simulink model "redundancy"  (R2020b)
settings: Solver=ode15s  StartTime=0.0  StopTime=T  MaxStep=0.01  RelTol=1e-3
values from neighbouring files (symbols this model uses):
  a1A = L1    (= 0.35)    [forward_kinematics_computation.m]
  a1B = L1    (= 0.35)    [forward_kinematics_computation.m]
  a2A = L2    (= 0.305)    [forward_kinematics_computation.m]
  a2B = L2    (= 0.305)    [forward_kinematics_computation.m]
  a3A = L3    (= 0.2662)    [forward_kinematics_computation.m]
  a3B = L3    (= 0.2662)    [forward_kinematics_computation.m]
  D = 1.047    [forward_kinematics_computation.m]
  dq0 = [0 0 0 0 0 0]'    [sim_redundancy.m]
  friction = [fv1p fv2p fv1A fv2A fv3A fv1B fv2B fv3B]    [sim_redundancy.m]
  g = [0 -g0 0]'    [sim_redundancy.m]
  Gd = diag([1000 1000 1000 1000 1000])    [sim_redundancy.m]
  Gd_nullspace = 10*eye(6)    [sim_redundancy.m]
  Gp = diag([3000 3000 3000 3000 1000])    [sim_redundancy.m]
  Gp_nullspace = 10*eye(6)    [sim_redundancy.m]
  info = struct('n_joints', n_joints,                'n_links', n_links,                'n_ee', n_ee,                'current_frame_index',    [1  2 3 4 5 6 7  8 9 10],                'previous_frame_index',   [0  1 2 3 4 2 6  7 5  8],                'next_frame_index',       [2 36 4 5 9 7 8 10 0  0],                'next_frame_type',        [0  1 0 0 0 0 0  0 0  0],                'previous_joint_index',  ...(+449 chars)    [sim_redundancy.m]
  Kd = 20*eye(6)    [sim_redundancy.m]
  Kp = 10*eye(6)    [sim_redundancy.m]
  L = 3.16 + 0.126    (= 3.286)    [forward_kinematics_computation.m]
  l1A = a1A/2    (= 0.175)    [forward_kinematics_computation.m]
  l1B = a1B/2    (= 0.175)    [forward_kinematics_computation.m]
  l2A = a2A/2    (= 0.1525)    [forward_kinematics_computation.m]
  l2B = a2B/2    (= 0.1525)    [forward_kinematics_computation.m]
  l3A = a3A/2    (= 0.1331)    [forward_kinematics_computation.m]
  l3B = a3B/2    (= 0.1331)    [forward_kinematics_computation.m]
  offA = -0.19    [forward_kinematics_computation.m]
  offB = 0.19    [forward_kinematics_computation.m]
  prova = 2    [sim_redundancy.m]
  q0 = [th1A_0 th2A_0 th3A_0 th1B_0 th2B_0 th3B_0]'    [sim_redundancy.m]
  qr = [0 -pi/3 pi/4 0 pi/4 pi/8]    [sim_redundancy.m]
  qr_ddot = zeros(1,6)    [sim_redundancy.m]
  qr_dot = zeros(1,6)    [sim_redundancy.m]
  th1A_0 = -pi/6    (= -0.523598775598)    [sim_redundancy.m]
  th1B_0 = pi/6    (= 0.523598775598)    [sim_redundancy.m]
  th2A_0 = pi/6    (= 0.523598775598)    [sim_redundancy.m]
  th2B_0 = -pi/6    (= -0.523598775598)    [sim_redundancy.m]
  th3A_0 = pi/6    (= 0.523598775598)    [sim_redundancy.m]
  th3B_0 = -pi/6    (= -0.523598775598)    [sim_redundancy.m]
  tipo_controllo = 1    [sim_redundancy.m]
  tipo_minimizzazione = 4    [sim_redundancy.m]
  x_ref = [-0.25 -0.8 0.19 -0.9 0]    [sim_redundancy.m]
  xddot_ref = [0 0 0 0 0]    [sim_redundancy.m]
  xdot_ref = [0 0 0 0 0]    [sim_redundancy.m]
undefined symbols (not defined in the file or in its folder): fv0, fv1A, fv1B, fv2A, fv2B, fv3A, fv3B, g0, Il1Azz, Il1Bzz, Il2Azz, Il2Bzz, Il3Azz, Il3Bzz, m_cables, m_crane, m_platform, ml1A, ml1B, ml2A, ml2B, ml3A, ml3B, X, Y, Z
libraries: sm_lib x137, nesl_utility x31
(part 1 of 5)
settings Model: Creator=giank  LastModifiedBy=giank
settings ExplorerConfigSet: InternalSimMechanicsExplorerSettings="<ExplorerConfiguration><canonicalview>default</canonicalview><AnimationSetting><BasePlaybackSpeed>1.0</BasePlaybackSpeed><PlaybackSpeedFactor>4.0</PlaybackSpeedFactor></AnimationSetting><TilePanel><TileInfo><Tiles Columns=\"1\" Count=\"1\" Rows=\"1\"><Column Weight=\"1\"/><Row Weight=\"1\"/><Tile Height=\"1\" Width=\"1\" X=\"0\" Y=\"0\"/></Tiles></TileInfo><SceneInfo><SceneViewer><BGColor><R>0.60000002384185791</R><G>0.60000002384185791</G><B>0.60000002384185791</B></BGColor><Camera><DoPerspective>off</DoPerspective><Position><X>8.32344120016426103e-09</X><Y>-2.30749996473441854</Y><Z>2.62102653220962445</Z></Position><Center><X>8.32344120016426103e-09</X><Y>-2.30749996473441854</Y><Z>6.6162316514351005e-08</Z></Center><Up><X>0</X><Y>1</Y><Z>-0</Z></Up><ViewLimDist>1</ViewLimDist><YLim>2.35612490177154532</YLim><XLim>3.05834251955443737</XLim></Camera></SceneViewer></SceneInfo></TilePanel><MechEditorPanel><Cameras/><GfxPanelCameraMap/><VideoCreator><PlaybackSpeedRatio>1.0</PlaybackSpeedRatio><FrameRate>30</FrameRate><VideoFormat>Motion JPEG AVI</VideoFormat><FrameSize>auto</FrameSize></VideoCreator></MechEditorPanel></ExplorerConfiguration>"

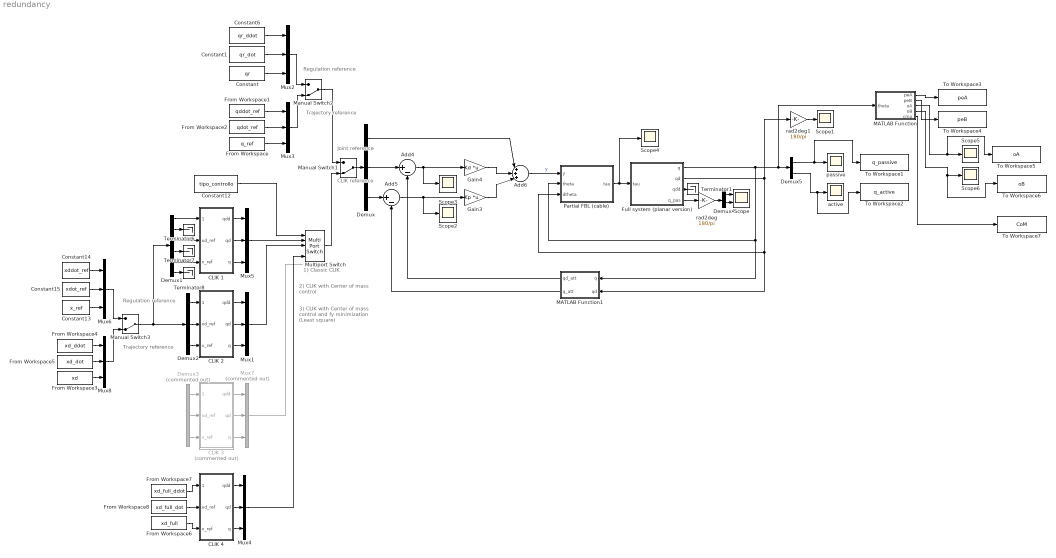
== system redundancy ==
  note: Regulation
      | reference
  note: CLIK
      | reference
  note: Trajectory
      | reference
  note: 3) CLIK with
      | Center of mass
      | control and
      | fy minimization
      | (Least square)
  note: 1) Classic
      | CLIK
  note: Trajectory
      | reference
  note: 2) CLIK with
      | Center of mass
      | control
  note: Joint
      | reference
  note: Regulation
      | reference
  Add4 : Sum  Inputs=|+-
  Add5 : Sum  Inputs=|+-
  Add6 : Sum  Inputs=|+++|
  CLIK 1 : Subsystem
  CLIK 2 : Subsystem
  CLIK 3 : Subsystem  Commented=on
  CLIK 4 : Subsystem
  Constant : Constant  Value=qr
  Constant1 : Constant  Value=qr_dot
  Constant12 : Constant  Value=tipo_controllo
  Constant13 : Constant  Value=x_ref
  Constant14 : Constant  Value=xddot_ref
  Constant15 : Constant  Value=xdot_ref
  Constant6 : Constant  Value=qr_ddot
  Demux : Demux  Outputs=3
  Demux1 : Demux  Outputs=[4 1 4 1 4 1]
  Demux2 : Demux  Outputs=[5 5 5]
  Demux3 : Demux  Commented=on  Outputs=[5 5 5]
  Demux4 : Demux  Outputs=2
  Demux5 : Demux  Outputs=[2 6]
  From Workspace : FromWorkspace  VariableName=q_ref
  From Workspace1 : FromWorkspace  VariableName=qddot_ref
  From Workspace2 : FromWorkspace  VariableName=qdot_ref
  From Workspace3 : FromWorkspace  VariableName=xd
  From Workspace4 : FromWorkspace  VariableName=xd_ddot
  From Workspace5 : FromWorkspace  VariableName=xd_dot
  From Workspace6 : FromWorkspace  VariableName=xd_full
  From Workspace7 : FromWorkspace  VariableName=xd_full_ddot
  From Workspace8 : FromWorkspace  VariableName=xd_full_dot
  Full system (planar version) : Subsystem
  Gain3 : Gain  Gain=Kp  Multiplication=Matrix(K*u)
  Gain4 : Gain  Gain=Kd  Multiplication=Matrix(K*u)
  MATLAB Function : MATLAB Function  TreatAsAtomicUnit=on
  MATLAB Function1 : MATLAB Function  TreatAsAtomicUnit=on
  Manual Switch1 : ManualSwitch  CurrentSetting=0
  Manual Switch2 : ManualSwitch  CurrentSetting=0
  Manual Switch3 : ManualSwitch  CurrentSetting=0
  Multiport Switch : MultiPortSwitch  DataPortOrder=Specify indices  DataPortIndices={1,2,3,4}
  Mux{1..6,8} (7 alike) : Mux  Inputs=3
  Mux7 : Mux  Commented=on  Inputs=3
  Partial FBL (cable) : MATLAB Function  TreatAsAtomicUnit=on
  Scope : Scope  NumInputPorts=2
  Scope{1..6} (6 alike) : Scope
  Terminator{1,6..8} (4 alike) : Terminator
  To Workspace1 : ToWorkspace  VariableName=q_passive  SaveFormat=Timeseries  SampleTime=-1
  To Workspace2 : ToWorkspace  VariableName=q_active  SaveFormat=Timeseries  SampleTime=-1
  To Workspace3 : ToWorkspace  VariableName=peA  SaveFormat=Timeseries  SampleTime=-1
  To Workspace4 : ToWorkspace  VariableName=peB  SaveFormat=Timeseries  SampleTime=-1
  To Workspace5 : ToWorkspace  VariableName=oA  SaveFormat=Timeseries  SampleTime=-1
  To Workspace6 : ToWorkspace  VariableName=oB  SaveFormat=Timeseries  SampleTime=-1
  To Workspace7 : ToWorkspace  VariableName=CoM  SaveFormat=Timeseries  SampleTime=-1
  active : Scope
  passive : Scope
  rad2deg : Gain  Gain=180/pi
  rad2deg1 : Gain  Gain=180/pi
  wires:
  Gain3/1 -> Add6/3
  Add6/1 -> Partial FBL (cable)/1(y)  "y"
  Demux/1 -> Add6/1
  Partial FBL (cable)/1(tau) -> Scope4/1, Full system (planar version)/1(tau)
  MATLAB Function1/1(qd_att) -> Add4/2
  Add4/1 -> Scope3/1, Gain4/1
  Add5/1 -> Gain3/1, Scope2/1
  Demux/2 -> Add4/1
  Full system (planar version)/3(qdd) -> Terminator1/1
  MATLAB Function1/2(q_att) -> Add5/2
  Full system (planar version)/1(q) -> MATLAB Function/1(theta), Demux5/1, Partial FBL (cable)/2(theta), MATLAB Function1/1(q)
  Demux/3 -> Add5/1
  Gain4/1 -> Add6/2
  Demux1/2 -> Terminator6/1
  Constant14/1 -> Mux6/1
  Mux6/1 -> Manual Switch3/1
  From Workspace3/1 -> Mux8/3
  From Workspace4/1 -> Mux8/1
  Constant12/1 -> Multiport Switch/1
  Multiport Switch/1 -> Manual Switch1/2
  From Workspace5/1 -> Mux8/2
  Constant13/1 -> Mux6/3
  Demux1/3 -> CLIK 1/2(xd_ref)
  Mux8/1 -> Manual Switch3/2
  Demux1/4 -> Terminator7/1
  Constant15/1 -> Mux6/2
  Demux1/5 -> CLIK 1/3(x_ref)
  Mux3/1 -> Manual Switch2/2
  Constant/1 -> Mux2/3
  Demux1/1 -> CLIK 1/1(xdd_ref)
  Demux1/6 -> Terminator8/1
  Manual Switch1/1 -> Demux/1
  Demux2/1 -> CLIK 2/1(xdd_ref)
  Constant6/1 -> Mux2/1
  Mux5/1 -> Multiport Switch/2
  Demux2/2 -> CLIK 2/2(xd_ref)
  Mux2/1 -> Manual Switch2/1
  CLIK 2/2(qd) -> Mux1/2
  CLIK 1/1(qdd) -> Mux5/1
  CLIK 1/2(qd) -> Mux5/2
  Manual Switch3/1 -> Demux1/1, Demux2/1
  Demux2/3 -> CLIK 2/3(x_ref)
  CLIK 2/1(qdd) -> Mux1/1
  From Workspace1/1 -> Mux3/1
  Manual Switch2/1 -> Manual Switch1/1
  Constant1/1 -> Mux2/2
  CLIK 2/3(q) -> Mux1/3
  Mux1/1 -> Multiport Switch/3
  From Workspace2/1 -> Mux3/2
  From Workspace/1 -> Mux3/3
  CLIK 1/3(q) -> Mux5/3
  Demux4/1 -> Scope/1
  Demux4/2 -> Scope/2
  rad2deg/1 -> Demux4/1
  Full system (planar version)/4(q_pas) -> rad2deg/1
  Demux3/2 -> CLIK 3/2(xd_ref)
  ? -> Demux3/1
  Mux7/1 -> ?
  CLIK 3/1(qdd) -> Mux7/1
  CLIK 3/3(q) -> Mux7/3
  CLIK 3/2(qd) -> Mux7/2
  Demux3/1 -> CLIK 3/1(xdd_ref)
  Demux3/3 -> CLIK 3/3(x_ref)
  Demux5/1 -> To Workspace1/1, passive/1
  Demux5/2 -> To Workspace2/1, active/1
  rad2deg1/1 -> Scope1/1
  Full system (planar version)/2(qd) -> rad2deg1/1, Partial FBL (cable)/3(dtheta), MATLAB Function1/2(qd)
  MATLAB Function/1(peA) -> To Workspace3/1
  MATLAB Function/2(peB) -> To Workspace4/1
  Mux4/1 -> Multiport Switch/5
  CLIK 4/1(qdd) -> Mux4/1
  CLIK 4/2(qd) -> Mux4/2
  CLIK 4/3(q) -> Mux4/3
  From Workspace7/1 -> CLIK 4/1(xdd_ref)
  From Workspace6/1 -> CLIK 4/3(x_ref)
  From Workspace8/1 -> CLIK 4/2(xd_ref)
  MATLAB Function/3(oA) -> To Workspace5/1, Scope5/1
  MATLAB Function/4(oB) -> To Workspace6/1, Scope6/1
  MATLAB Function/5(cmx) -> To Workspace7/1

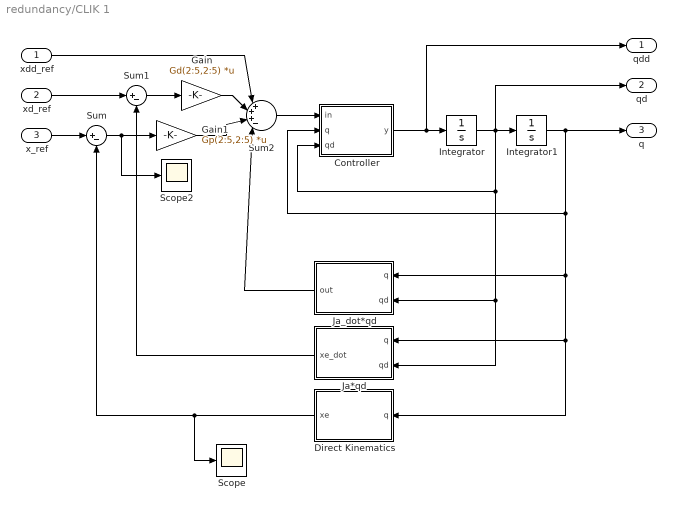
== system redundancy/CLIK 1 ==
  xdd_ref : Inport
  xd_ref : Inport  Port=2
  x_ref : Inport  Port=3
  Controller : MATLAB Function  TreatAsAtomicUnit=on
  Direct Kinematics : MATLAB Function  TreatAsAtomicUnit=on
  Gain : Gain  Gain=Gd(2:5,2:5)  Multiplication=Matrix(K*u)
  Gain1 : Gain  Gain=Gp(2:5,2:5)  Multiplication=Matrix(K*u)
  Integrator : Integrator  InitialCondition=dq0
  Integrator1 : Integrator  InitialCondition=q0
  Ja*qd : MATLAB Function  TreatAsAtomicUnit=on
  Ja_dot*qd : MATLAB Function  TreatAsAtomicUnit=on
  Scope : Scope
  Scope2 : Scope
  Sum : Sum  Inputs=|+-
  Sum1 : Sum  Inputs=|+-
  Sum2 : Sum  Inputs=|+++-|
  qdd : Outport
  qd : Outport  Port=2
  q : Outport  Port=3
  wires:
  Controller/1(y) -> qdd/1, Integrator/1
  Sum1/1 -> Gain/1
  Direct Kinematics/1(xe) -> Scope/1, Sum/2
  Gain/1 -> Sum2/2
  Integrator/1 -> qd/1, Integrator1/1, Controller/3(qd), Ja_dot*qd/2(qd), Ja*qd/2(qd)
  Ja*qd/1(xe_dot) -> Sum1/2
  Gain1/1 -> Sum2/3
  Integrator1/1 -> q/1, Ja_dot*qd/1(q), Ja*qd/1(q), Direct Kinematics/1(q), Controller/2(q)
  Sum2/1 -> Controller/1(in)
  Sum/1 -> Scope2/1, Gain1/1
  Ja_dot*qd/1(out) -> Sum2/4
  x_ref/1 -> Sum/1
  xd_ref/1 -> Sum1/1
  xdd_ref/1 -> Sum2/1

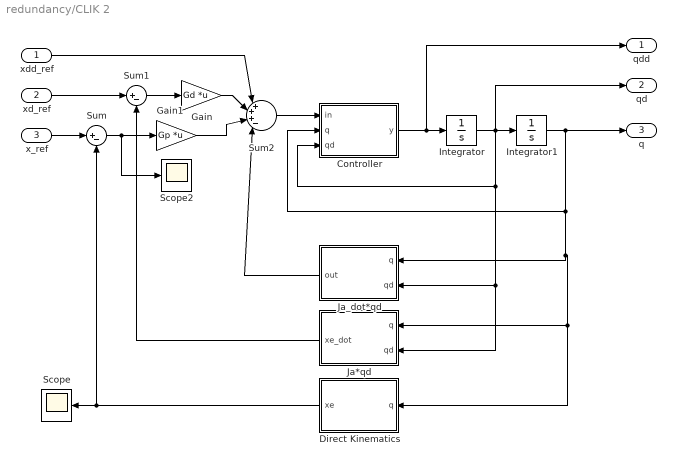
== system redundancy/CLIK 2 ==
  xdd_ref : Inport
  xd_ref : Inport  Port=2
  x_ref : Inport  Port=3
  Controller : MATLAB Function  TreatAsAtomicUnit=on
  Direct Kinematics : MATLAB Function  TreatAsAtomicUnit=on
  Gain : Gain  Gain=Gd  Multiplication=Matrix(K*u)
  Gain1 : Gain  Gain=Gp  Multiplication=Matrix(K*u)
  Integrator : Integrator  InitialCondition=dq0
  Integrator1 : Integrator  InitialCondition=q0
  Ja*qd : MATLAB Function  TreatAsAtomicUnit=on
  Ja_dot*qd : MATLAB Function  TreatAsAtomicUnit=on
  Scope : Scope
  Scope2 : Scope
  Sum : Sum  Inputs=|+-
  Sum1 : Sum  Inputs=|+-
  Sum2 : Sum  Inputs=|+++-|
  qdd : Outport
  qd : Outport  Port=2
  q : Outport  Port=3
  wires:
  Controller/1(y) -> qdd/1, Integrator/1
  Sum1/1 -> Gain/1
  Direct Kinematics/1(xe) -> Scope/1, Sum/2
  Gain/1 -> Sum2/2
  Integrator/1 -> Ja*qd/2(qd), Ja_dot*qd/2(qd), Controller/3(qd), qd/1, Integrator1/1
  Ja*qd/1(xe_dot) -> Sum1/2
  Gain1/1 -> Sum2/3
  Integrator1/1 -> Ja_dot*qd/1(q), Direct Kinematics/1(q), Ja*qd/1(q), Controller/2(q), q/1
  Sum2/1 -> Controller/1(in)
  Sum/1 -> Scope2/1, Gain1/1
  Ja_dot*qd/1(out) -> Sum2/4
  x_ref/1 -> Sum/1
  xd_ref/1 -> Sum1/1
  xdd_ref/1 -> Sum2/1

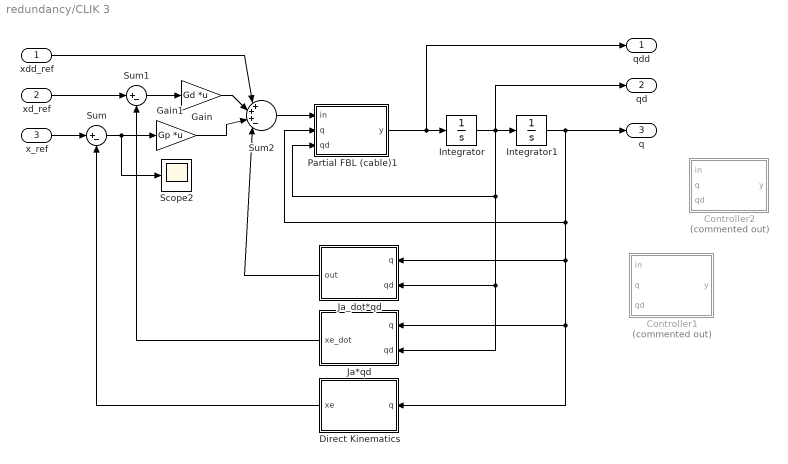
== system redundancy/CLIK 3 ==
  xdd_ref : Inport
  xd_ref : Inport  Port=2
  x_ref : Inport  Port=3
  Controller1 : MATLAB Function  Commented=on  TreatAsAtomicUnit=on
  Controller2 : MATLAB Function  Commented=on  TreatAsAtomicUnit=on
  Direct Kinematics : MATLAB Function  TreatAsAtomicUnit=on
  Gain : Gain  Gain=Gd  Multiplication=Matrix(K*u)
  Gain1 : Gain  Gain=Gp  Multiplication=Matrix(K*u)
  Integrator : Integrator  InitialCondition=dq0
  Integrator1 : Integrator  InitialCondition=q0
  Ja*qd : MATLAB Function  TreatAsAtomicUnit=on
  Ja_dot*qd : MATLAB Function  TreatAsAtomicUnit=on
  Partial FBL (cable)1 : MATLAB Function  TreatAsAtomicUnit=on
  Scope2 : Scope
  Sum : Sum  Inputs=|+-
  Sum1 : Sum  Inputs=|+-
  Sum2 : Sum  Inputs=|+++-|
  qdd : Outport
  qd : Outport  Port=2
  q : Outport  Port=3
  wires:
  Partial FBL (cable)1/1(y) -> qdd/1, Integrator/1
  Sum1/1 -> Gain/1
  Direct Kinematics/1(xe) -> Sum/2
  Gain/1 -> Sum2/2
  Integrator/1 -> Partial FBL (cable)1/3(qd), Ja*qd/2(qd), Ja_dot*qd/2(qd), qd/1, Integrator1/1
  Ja*qd/1(xe_dot) -> Sum1/2
  Gain1/1 -> Sum2/3
  Integrator1/1 -> Partial FBL (cable)1/2(q), Direct Kinematics/1(q), Ja*qd/1(q), Ja_dot*qd/1(q), q/1
  Sum2/1 -> Partial FBL (cable)1/1(in)
  Sum/1 -> Scope2/1, Gain1/1
  Ja_dot*qd/1(out) -> Sum2/4
  x_ref/1 -> Sum/1
  xd_ref/1 -> Sum1/1
  xdd_ref/1 -> Sum2/1

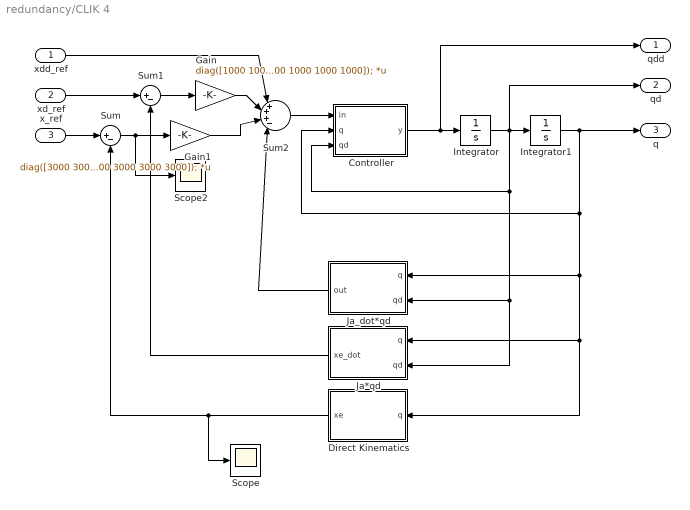
== system redundancy/CLIK 4 ==
  xdd_ref : Inport
  xd_ref : Inport  Port=2
  x_ref : Inport  Port=3
  Controller : MATLAB Function  TreatAsAtomicUnit=on
  Direct Kinematics : MATLAB Function  TreatAsAtomicUnit=on
  Gain : Gain  Gain=diag([1000 1000 1000 1000 1000 1000]);  Multiplication=Matrix(K*u)
  Gain1 : Gain  Gain=diag([3000 3000 3000 3000 3000 3000]);  Multiplication=Matrix(K*u)
  Integrator : Integrator  InitialCondition=dq0
  Integrator1 : Integrator  InitialCondition=q0
  Ja*qd : MATLAB Function  TreatAsAtomicUnit=on
  Ja_dot*qd : MATLAB Function  TreatAsAtomicUnit=on
  Scope : Scope
  Scope2 : Scope
  Sum : Sum  Inputs=|+-
  Sum1 : Sum  Inputs=|+-
  Sum2 : Sum  Inputs=|+++-|
  qdd : Outport
  qd : Outport  Port=2
  q : Outport  Port=3
  wires:
  Controller/1(y) -> qdd/1, Integrator/1
  Sum1/1 -> Gain/1
  Direct Kinematics/1(xe) -> Scope/1, Sum/2
  Gain/1 -> Sum2/2
  Integrator/1 -> qd/1, Integrator1/1, Controller/3(qd), Ja_dot*qd/2(qd), Ja*qd/2(qd)
  Ja*qd/1(xe_dot) -> Sum1/2
  Gain1/1 -> Sum2/3
  Integrator1/1 -> q/1, Ja_dot*qd/1(q), Ja*qd/1(q), Direct Kinematics/1(q), Controller/2(q)
  Sum2/1 -> Controller/1(in)
  Sum/1 -> Scope2/1, Gain1/1
  Ja_dot*qd/1(out) -> Sum2/4
  x_ref/1 -> Sum/1
  xd_ref/1 -> Sum1/1
  xdd_ref/1 -> Sum2/1

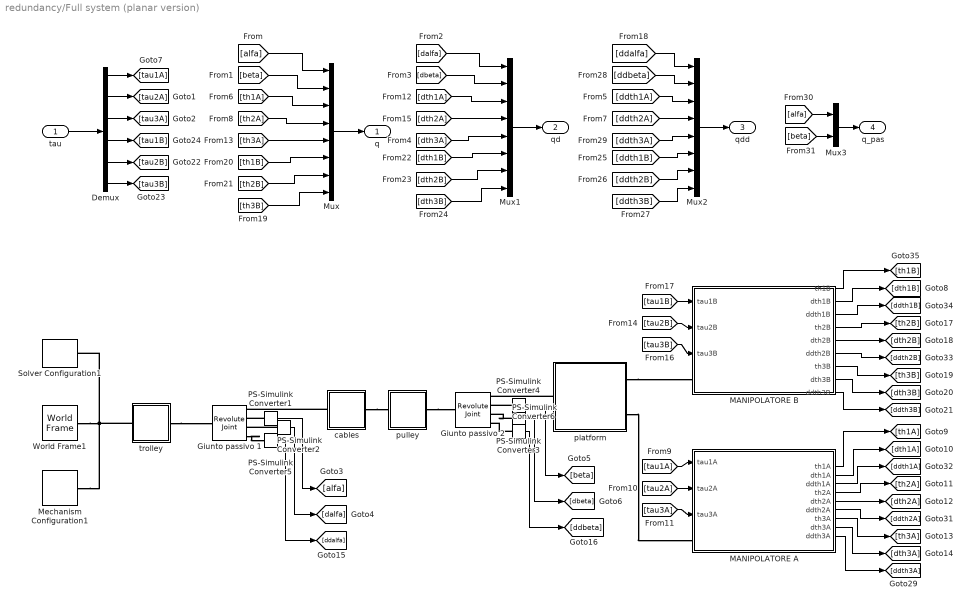
== system redundancy/Full system (planar version) ==
  tau : Inport
  Demux : Demux  Outputs=6
  Giunto passivo 1 : sm_lib/Joints/Revolute Joint  JointMode=Normal  SenseConstraintForce=off  SenseConstraintForceX=off  SenseConstraintForceY=off  SenseConstraintForceZ=off  SenseConstraintTorque=off  SenseConstraintTorqueX=off  SenseConstraintTorqueY=off  SenseConstraintTorqueZ=off  SenseTotalForce=off  SenseTotalForceX=off  SenseTotalForceY=off  SenseTotalForceZ=off  SenseTotalTorque=off  SenseTotalTorqueX=off  SenseTotalTorqueY=off  SenseTotalTorqueZ=off  CompositeWrenchDir=FollowerOnBase  CompositeWrenchFrame=BaseFrame  EquilibriumPosition=0  EquilibriumPositionUnits=deg  SpringStiffness=0  SpringStiffnessUnits=N*m/deg  DampingCoefficient=fv1p  DampingCoefficientUnits=N*m/(rad/s)  TorqueActuationMode=NoTorque  MotionActuationMode=ComputedMotion  SensePosition=on  SenseVelocity=on  SenseAcceleration=on  SenseTorqueForce=off  SenseLowerLimitTorqueForce=off  SenseUpperLimitTorqueForce=off  LowerLimitSpecify=off  LowerLimitBound=-90  LowerLimitBoundUnits=deg  LowerLimitStiffness=1e4  LowerLimitStiffnessUnits=N*m/deg  LowerLimitDamping=10  LowerLimitDampingUnits=N*m/(deg/s)  LowerLimitTransitionRegionWidth=0.1  LowerLimitTransitionRegionWidthUnits=deg  UpperLimitSpecify=off  UpperLimitBound=90  UpperLimitBoundUnits=deg  UpperLimitStiffness=1e4  UpperLimitStiffnessUnits=N*m/deg  UpperLimitDamping=10  UpperLimitDampingUnits=N*m/(deg/s)  UpperLimitTransitionRegionWidth=0.1  UpperLimitTransitionRegionWidthUnits=deg  PositionTargetSpecify=on  PositionTargetPriority=High  PositionTargetValue=alfa_0  PositionTargetValueUnits=rad  VelocityTargetSpecify=off  VelocityTargetPriority=High  VelocityTargetValue=0  VelocityTargetValueUnits=deg/s
  Giunto passivo 2 : sm_lib/Joints/Revolute Joint  JointMode=Normal  SenseConstraintForce=off  SenseConstraintForceX=off  SenseConstraintForceY=off  SenseConstraintForceZ=off  SenseConstraintTorque=off  SenseConstraintTorqueX=off  SenseConstraintTorqueY=off  SenseConstraintTorqueZ=off  SenseTotalForce=off  SenseTotalForceX=off  SenseTotalForceY=off  SenseTotalForceZ=off  SenseTotalTorque=off  SenseTotalTorqueX=off  SenseTotalTorqueY=off  SenseTotalTorqueZ=off  CompositeWrenchDir=FollowerOnBase  CompositeWrenchFrame=BaseFrame  EquilibriumPosition=0  EquilibriumPositionUnits=deg  SpringStiffness=0  SpringStiffnessUnits=N*m/deg  DampingCoefficient=fv2p  DampingCoefficientUnits=N*m/(rad/s)  TorqueActuationMode=NoTorque  MotionActuationMode=ComputedMotion  SensePosition=on  SenseVelocity=on  SenseAcceleration=on  SenseTorqueForce=off  SenseLowerLimitTorqueForce=off  SenseUpperLimitTorqueForce=off  LowerLimitSpecify=off  LowerLimitBound=-90  LowerLimitBoundUnits=deg  LowerLimitStiffness=1e4  LowerLimitStiffnessUnits=N*m/deg  LowerLimitDamping=10  LowerLimitDampingUnits=N*m/(deg/s)  LowerLimitTransitionRegionWidth=0.1  LowerLimitTransitionRegionWidthUnits=deg  UpperLimitSpecify=off  UpperLimitBound=90  UpperLimitBoundUnits=deg  UpperLimitStiffness=1e4  UpperLimitStiffnessUnits=N*m/deg  UpperLimitDamping=10  UpperLimitDampingUnits=N*m/(deg/s)  UpperLimitTransitionRegionWidth=0.1  UpperLimitTransitionRegionWidthUnits=deg  PositionTargetSpecify=on  PositionTargetPriority=High  PositionTargetValue=beta_0  PositionTargetValueUnits=rad  VelocityTargetSpecify=off  VelocityTargetPriority=High  VelocityTargetValue=0  VelocityTargetValueUnits=deg/s
  MANIPOLATORE A : Subsystem  mask{th1_0=th1A_0, th2_0=th2A_0, th3_0=th3A_0, fv1=fv1A, fv2=fv2A, fv3=fv3A, a1=a1A, a2=a2A, a3=a3A, ml1=ml1A, ml2=ml2A, ml3=ml3A}
      mask prompts: th1_0 "th1_0 (rad)"; th2_0 "th2_0 (rad)"; th3_0 "th3_0 (rad)"; fv1 "Damping coeff. joint 1 (N*m/(rad/s))"; fv2 "Damping coeff. joint 2 (N*m/(rad/s))"; fv3 "Damping coeff. joint 3 (N*m/(rad/s))"; a1 "a1 (m)"; a2 "a2 (m)"; a3 "a3 (m)"; ml1 "ml1 (kg)"; ml2 "ml2 (kg)"; ml3 "ml3 (kg)"
  MANIPOLATORE B : Subsystem  mask{th1_0=th1B_0, th2_0=th2B_0, th3_0=th3B_0, fv1=fv1B, fv2=fv2B, fv3=fv3B, a1=a1B, a2=a2B, a3=a3B, ml1=ml1B, ml2=ml2B, ml3=ml3B}
      mask prompts: th1_0 "th1_0 (rad)"; th2_0 "th2_0 (rad)"; th3_0 "th3_0 (rad)"; fv1 "Damping coeff. joint 1 (N*m/(rad/s))"; fv2 "Damping coeff. joint 2 (N*m/(rad/s))"; fv3 "Damping coeff. joint 3 (N*m/(rad/s))"; a1 "a1 (m)"; a2 "a2 (m)"; a3 "a3 (m)"; ml1 "ml1 (kg)"; ml2 "ml2 (kg)"; ml3 "ml3 (kg)"
  Mechanism Configuration1 : sm_lib/Utilities/Mechanism Configuration  UniformGravity=Constant  GravityVector=[0 -9.81 0]  GravityVectorUnits=m/s^2  GravityUnits=m/s^2  LinearizationDelta=0.001  JointModeTransitionNonlinearIterations=2
  Mux : Mux  Inputs=8
  Mux1 : Mux  Inputs=8
  Mux2 : Mux  Inputs=8
  Mux3 : Mux  Inputs=2
  PS-Simulink Converter{1..6} (6 alike) : nesl_utility/PS-Simulink Converter  PhysicalDomain=network_engine_domain  SubClassName=ps_output  LeftPortType=input  RightPortType=output  PseudoPeriodic=off  Frequencies=[]  Unit=inherit  AffineConversion=off
  Solver Configuration1 : nesl_utility/Solver Configuration  PhysicalDomain=network_engine_domain  SubClassName=solver  LeftPortType=input  RightPortType=generic  Tones=[]  Harmonics=[]  SimulateNoise=off  Profile=off  UseLocalSampling=off  EnableSwitchedLinearOptims=on  FrequencyDomain=off  UseCCode=off  RelTol=0.001  AbsTol=1e-06  MinStep=1e-09  ToWorkspace=off  RevertToSquareIcSolve=off  NumHomotopyIterations=100  PhasorMode=off  PhasorModeNumHarmonics=1  DoDC=off  ResidualTolerance=1e-09  UseLocalSolver=off  LocalSolverChoice=NE_BACKWARD_EULER_ADVANCER  LocalSolverSampleTime=0.001  DoFixedCost=off  MaxNonlinIter=3  MaxModeIter=2  ComputeImpulses=off  ImpulseIterations=2  LinearAlgebra=Sparse  EquationFormulation=NE_TIME_EF  DelaysMemoryBudget=1024  AutomaticFiltering=on  FilteringTimeConstant=0.001  PartitionStorageMethod=AS_NEEDED  PartitionMemoryBudget=1024  PartitionMethod=FAST
  World Frame1 : sm_lib/Frames and Transforms/World Frame
  cables : Subsystem
  platform : Subsystem
  pulley : Subsystem
  trolley : Subsystem
  q : Outport
  qd : Outport  Port=2
  qdd : Outport  Port=3
  q_pas : Outport  Port=4
  wires:
  Mux/1 -> q/1
  PS-Simulink Converter1/1 -> [alfa]
  PS-Simulink Converter2/1 -> [dalfa]
  PS-Simulink Converter4/1 -> [beta]
  PS-Simulink Converter3/1 -> [dbeta]
  tau/1 -> Demux/1
  Mux1/1 -> qd/1
  Demux/1 -> [tau1A]
  Demux/3 -> [tau3A]
  Demux/2 -> [tau2A]
  Demux/4 -> [tau1B]
  Demux/5 -> [tau2B]
  [beta] -> Mux/2
  [alfa] -> Mux/1
  [th1A] -> Mux/3
  [th2A] -> Mux/4
  [th3A] -> Mux/5
  [th1B] -> Mux/6
  [th2B] -> Mux/7
  [th3B] -> Mux/8
  [dalfa] -> Mux1/1
  [dbeta] -> Mux1/2
  [dth1A] -> Mux1/3
  [dth2A] -> Mux1/4
  [dth3A] -> Mux1/5
  [dth1B] -> Mux1/6
  [dth2B] -> Mux1/7
  [dth3B] -> Mux1/8
  Demux/6 -> [tau3B]
  PS-Simulink Converter5/1 -> [ddalfa]
  PS-Simulink Converter6/1 -> [ddbeta]
  [ddalfa] -> Mux2/1
  Mux2/1 -> qdd/1
  [ddth1A] -> Mux2/3
  [ddth3B] -> Mux2/8
  [ddth2B] -> Mux2/7
  [ddth2A] -> Mux2/4
  [ddbeta] -> Mux2/2
  [ddth1B] -> Mux2/6
  [ddth3A] -> Mux2/5
  [alfa] -> Mux3/1
  [beta] -> Mux3/2
  Mux3/1 -> q_pas/1
  MANIPOLATORE A/1(th1A) -> [th1A]
  [tau3B] -> MANIPOLATORE B/3(tau3B)
  MANIPOLATORE B/1(th1B) -> [th1B]
  [tau1B] -> MANIPOLATORE B/1(tau1B)
  [tau2B] -> MANIPOLATORE B/2(tau2B)
  MANIPOLATORE B/4(th2B) -> [th2B]
  MANIPOLATORE B/5(dth2B) -> [dth2B]
  MANIPOLATORE B/7(th3B) -> [th3B]
  MANIPOLATORE A/5(dth2A) -> [dth2A]
  [tau2A] -> MANIPOLATORE A/2(tau2A)
  MANIPOLATORE A/4(th2A) -> [th2A]
  MANIPOLATORE A/8(dth3A) -> [dth3A]
  MANIPOLATORE A/9(ddth3A) -> [ddth3A]
  MANIPOLATORE B/6(ddth2B) -> [ddth2B]
  [tau1A] -> MANIPOLATORE A/1(tau1A)
  MANIPOLATORE A/7(th3A) -> [th3A]
  MANIPOLATORE B/8(dth3B) -> [dth3B]
  MANIPOLATORE B/9(ddth3B) -> [ddth3B]
  MANIPOLATORE A/2(dth1A) -> [dth1A]
  MANIPOLATORE A/6(ddth2A) -> [ddth2A]
  [tau3A] -> MANIPOLATORE A/3(tau3A)
  MANIPOLATORE B/2(dth1B) -> [dth1B]
  MANIPOLATORE B/3(ddth1B) -> [ddth1B]
  MANIPOLATORE A/3(ddth1A) -> [ddth1A]
  connections:
  Mechanism Configuration1/RConn1 -- trolley/LConn1 -- World Frame1/RConn1 -- Solver Configuration1/RConn1
  cables/LConn1 -- Giunto passivo 1/RConn1
  trolley/RConn1 -- Giunto passivo 1/LConn1
  platform/LConn1 -- Giunto passivo 2/RConn1
  PS-Simulink Converter1/LConn1 -- Giunto passivo 1/RConn2
  PS-Simulink Converter4/LConn1 -- Giunto passivo 2/RConn2
  PS-Simulink Converter3/LConn1 -- Giunto passivo 2/RConn3
  PS-Simulink Converter2/LConn1 -- Giunto passivo 1/RConn3
  Giunto passivo 1/RConn4 -- PS-Simulink Converter5/LConn1
  PS-Simulink Converter6/LConn1 -- Giunto passivo 2/RConn4
  platform/RConn1 -- MANIPOLATORE B/LConn1
  platform/RConn2 -- MANIPOLATORE A/LConn1
  cables/RConn1 -- pulley/LConn1
  pulley/RConn1 -- Giunto passivo 2/LConn1

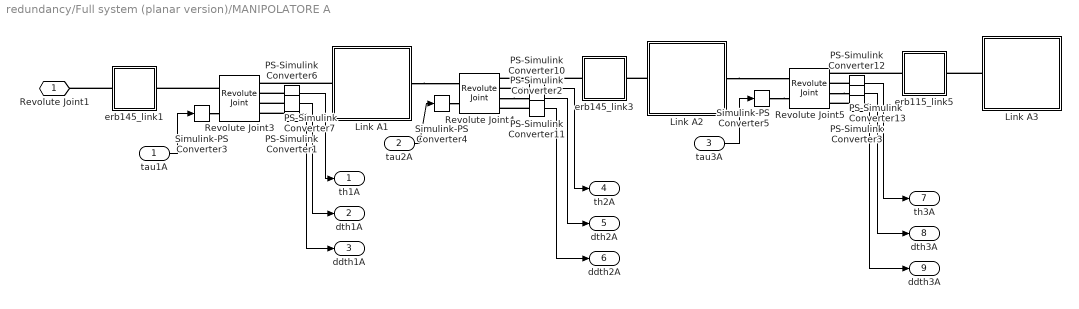
== system redundancy/Full system (planar version)/MANIPOLATORE A ==
  tau1A : Inport
  tau2A : Inport  Port=2
  tau3A : Inport  Port=3
  Link A1 : Subsystem
  Link A2 : Subsystem
  Link A3 : Subsystem
  PS-Simulink Converter{1..3,6..7,10..13} (9 alike) : nesl_utility/PS-Simulink Converter  PhysicalDomain=network_engine_domain  SubClassName=ps_output  LeftPortType=input  RightPortType=output  PseudoPeriodic=off  Frequencies=[]  Unit=inherit  AffineConversion=off
  Revolute Joint3 : sm_lib/Joints/Revolute Joint  JointMode=Normal  SenseConstraintForce=off  SenseConstraintForceX=off  SenseConstraintForceY=off  SenseConstraintForceZ=off  SenseConstraintTorque=off  SenseConstraintTorqueX=off  SenseConstraintTorqueY=off  SenseConstraintTorqueZ=off  SenseTotalForce=off  SenseTotalForceX=off  SenseTotalForceY=off  SenseTotalForceZ=off  SenseTotalTorque=off  SenseTotalTorqueX=off  SenseTotalTorqueY=off  SenseTotalTorqueZ=off  CompositeWrenchDir=FollowerOnBase  CompositeWrenchFrame=BaseFrame  EquilibriumPosition=0  EquilibriumPositionUnits=deg  SpringStiffness=0  SpringStiffnessUnits=N*m/deg  DampingCoefficient=fv1  DampingCoefficientUnits=N*m/(rad/s)  TorqueActuationMode=InputTorque  MotionActuationMode=ComputedMotion  SensePosition=on  SenseVelocity=on  SenseAcceleration=on  SenseTorqueForce=off  SenseLowerLimitTorqueForce=off  SenseUpperLimitTorqueForce=off  LowerLimitSpecify=off  LowerLimitBound=-90  LowerLimitBoundUnits=deg  LowerLimitStiffness=1e4  LowerLimitStiffnessUnits=N*m/deg  LowerLimitDamping=10  LowerLimitDampingUnits=N*m/(deg/s)  LowerLimitTransitionRegionWidth=0.1  LowerLimitTransitionRegionWidthUnits=deg  UpperLimitSpecify=off  UpperLimitBound=90  UpperLimitBoundUnits=deg  UpperLimitStiffness=1e4  UpperLimitStiffnessUnits=N*m/deg  UpperLimitDamping=10  UpperLimitDampingUnits=N*m/(deg/s)  UpperLimitTransitionRegionWidth=0.1  UpperLimitTransitionRegionWidthUnits=deg  PositionTargetSpecify=on  PositionTargetPriority=High  PositionTargetValue=th1_0  PositionTargetValueUnits=rad  VelocityTargetSpecify=off  VelocityTargetPriority=High  VelocityTargetValue=0  VelocityTargetValueUnits=deg/s
  Revolute Joint4 : sm_lib/Joints/Revolute Joint  JointMode=Normal  SenseConstraintForce=off  SenseConstraintForceX=off  SenseConstraintForceY=off  SenseConstraintForceZ=off  SenseConstraintTorque=off  SenseConstraintTorqueX=off  SenseConstraintTorqueY=off  SenseConstraintTorqueZ=off  SenseTotalForce=off  SenseTotalForceX=off  SenseTotalForceY=off  SenseTotalForceZ=off  SenseTotalTorque=off  SenseTotalTorqueX=off  SenseTotalTorqueY=off  SenseTotalTorqueZ=off  CompositeWrenchDir=FollowerOnBase  CompositeWrenchFrame=BaseFrame  EquilibriumPosition=0  EquilibriumPositionUnits=deg  SpringStiffness=0  SpringStiffnessUnits=N*m/deg  DampingCoefficient=fv2  DampingCoefficientUnits=N*m/(rad/s)  TorqueActuationMode=InputTorque  MotionActuationMode=ComputedMotion  SensePosition=on  SenseVelocity=on  SenseAcceleration=on  SenseTorqueForce=off  SenseLowerLimitTorqueForce=off  SenseUpperLimitTorqueForce=off  LowerLimitSpecify=off  LowerLimitBound=-90  LowerLimitBoundUnits=deg  LowerLimitStiffness=1e4  LowerLimitStiffnessUnits=N*m/deg  LowerLimitDamping=10  LowerLimitDampingUnits=N*m/(deg/s)  LowerLimitTransitionRegionWidth=0.1  LowerLimitTransitionRegionWidthUnits=deg  UpperLimitSpecify=off  UpperLimitBound=90  UpperLimitBoundUnits=deg  UpperLimitStiffness=1e4  UpperLimitStiffnessUnits=N*m/deg  UpperLimitDamping=10  UpperLimitDampingUnits=N*m/(deg/s)  UpperLimitTransitionRegionWidth=0.1  UpperLimitTransitionRegionWidthUnits=deg  PositionTargetSpecify=on  PositionTargetPriority=High  PositionTargetValue=th2_0  PositionTargetValueUnits=rad  VelocityTargetSpecify=off  VelocityTargetPriority=High  VelocityTargetValue=0  VelocityTargetValueUnits=deg/s
  Revolute Joint5 : sm_lib/Joints/Revolute Joint  JointMode=Normal  SenseConstraintForce=off  SenseConstraintForceX=off  SenseConstraintForceY=off  SenseConstraintForceZ=off  SenseConstraintTorque=off  SenseConstraintTorqueX=off  SenseConstraintTorqueY=off  SenseConstraintTorqueZ=off  SenseTotalForce=off  SenseTotalForceX=off  SenseTotalForceY=off  SenseTotalForceZ=off  SenseTotalTorque=off  SenseTotalTorqueX=off  SenseTotalTorqueY=off  SenseTotalTorqueZ=off  CompositeWrenchDir=FollowerOnBase  CompositeWrenchFrame=BaseFrame  EquilibriumPosition=0  EquilibriumPositionUnits=deg  SpringStiffness=0  SpringStiffnessUnits=N*m/deg  DampingCoefficient=fv3  DampingCoefficientUnits=N*m/(rad/s)  TorqueActuationMode=InputTorque  MotionActuationMode=ComputedMotion  SensePosition=on  SenseVelocity=on  SenseAcceleration=on  SenseTorqueForce=off  SenseLowerLimitTorqueForce=off  SenseUpperLimitTorqueForce=off  LowerLimitSpecify=off  LowerLimitBound=-90  LowerLimitBoundUnits=deg  LowerLimitStiffness=1e4  LowerLimitStiffnessUnits=N*m/deg  LowerLimitDamping=10  LowerLimitDampingUnits=N*m/(deg/s)  LowerLimitTransitionRegionWidth=0.1  LowerLimitTransitionRegionWidthUnits=deg  UpperLimitSpecify=off  UpperLimitBound=90  UpperLimitBoundUnits=deg  UpperLimitStiffness=1e4  UpperLimitStiffnessUnits=N*m/deg  UpperLimitDamping=10  UpperLimitDampingUnits=N*m/(deg/s)  UpperLimitTransitionRegionWidth=0.1  UpperLimitTransitionRegionWidthUnits=deg  PositionTargetSpecify=on  PositionTargetPriority=High  PositionTargetValue=th3_0  PositionTargetValueUnits=rad  VelocityTargetSpecify=off  VelocityTargetPriority=High  VelocityTargetValue=0  VelocityTargetValueUnits=deg/s
  Simulink-PS Converter3 : nesl_utility/Simulink-PS Converter  PhysicalDomain=network_engine_domain  SubClassName=ps_input  LeftPortType=input  RightPortType=output  PseudoPeriodic=off  Frequencies=[]  NoiseDistribution=none  NoiseParameters=[]  Unit=1  AffineConversion=off  FilteringAndDerivatives=provide  SimscapeFilterOrder=1  InputFilterTimeConstant=0.001  UdotUserProvided=0
  Simulink-PS Converter4 : nesl_utility/Simulink-PS Converter  PhysicalDomain=network_engine_domain  SubClassName=ps_input  LeftPortType=input  RightPortType=output  PseudoPeriodic=off  Frequencies=[]  NoiseDistribution=none  NoiseParameters=[]  Unit=1  AffineConversion=off  FilteringAndDerivatives=provide  SimscapeFilterOrder=1  InputFilterTimeConstant=0.001  UdotUserProvided=0
  Simulink-PS Converter5 : nesl_utility/Simulink-PS Converter  PhysicalDomain=network_engine_domain  SubClassName=ps_input  LeftPortType=input  RightPortType=output  PseudoPeriodic=off  Frequencies=[]  NoiseDistribution=none  NoiseParameters=[]  Unit=1  AffineConversion=off  FilteringAndDerivatives=provide  SimscapeFilterOrder=1  InputFilterTimeConstant=0.001  UdotUserProvided=0
  erb115_link5 : Subsystem
  erb145_link1 : Subsystem
  erb145_link3 : Subsystem
  Revolute Joint1 : PMIOPort  Side=Left
  th1A : Outport
  dth1A : Outport  Port=2
  ddth1A : Outport  Port=3
  th2A : Outport  Port=4
  dth2A : Outport  Port=5
  ddth2A : Outport  Port=6
  th3A : Outport  Port=7
  dth3A : Outport  Port=8
  ddth3A : Outport  Port=9
  wires:
  PS-Simulink Converter11/1 -> dth2A/1
  PS-Simulink Converter12/1 -> th3A/1
  PS-Simulink Converter13/1 -> dth3A/1
  tau1A/1 -> Simulink-PS Converter3/1
  tau3A/1 -> Simulink-PS Converter5/1
  tau2A/1 -> Simulink-PS Converter4/1
  PS-Simulink Converter10/1 -> th2A/1
  PS-Simulink Converter6/1 -> th1A/1
  PS-Simulink Converter7/1 -> dth1A/1
  PS-Simulink Converter1/1 -> ddth1A/1
  PS-Simulink Converter2/1 -> ddth2A/1
  PS-Simulink Converter3/1 -> ddth3A/1
  connections:
  PS-Simulink Converter12/LConn1 -- Revolute Joint5/RConn2
  Link A2/RConn1 -- Revolute Joint5/LConn1
  PS-Simulink Converter6/LConn1 -- Revolute Joint3/RConn2
  Revolute Joint4/RConn3 -- PS-Simulink Converter11/LConn1
  Link A1/RConn1 -- Revolute Joint4/LConn1
  Simulink-PS Converter5/RConn1 -- Revolute Joint5/LConn2
  PS-Simulink Converter7/LConn1 -- Revolute Joint3/RConn3
  Simulink-PS Converter4/RConn1 -- Revolute Joint4/LConn2
  Link A1/LConn1 -- Revolute Joint3/RConn1
  Revolute Joint3/LConn1 -- erb145_link1/RConn1
  erb145_link3/LConn1 -- Revolute Joint4/RConn1
  Revolute Joint5/RConn3 -- PS-Simulink Converter13/LConn1
  erb115_link5/LConn1 -- Revolute Joint5/RConn1
  Simulink-PS Converter3/RConn1 -- Revolute Joint3/LConn2
  PS-Simulink Converter10/LConn1 -- Revolute Joint4/RConn2
  PS-Simulink Converter1/LConn1 -- Revolute Joint3/RConn4
  PS-Simulink Converter2/LConn1 -- Revolute Joint4/RConn4
  PS-Simulink Converter3/LConn1 -- Revolute Joint5/RConn4
  erb145_link1/LConn1 -- Revolute Joint1/RConn1
  Link A2/LConn1 -- erb145_link3/RConn1
  Link A3/LConn1 -- erb115_link5/RConn1

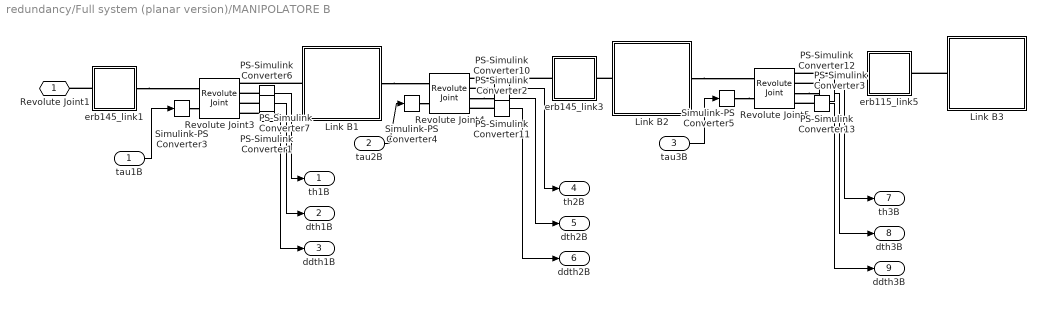
== system redundancy/Full system (planar version)/MANIPOLATORE B ==
  tau1B : Inport
  tau2B : Inport  Port=2
  tau3B : Inport  Port=3
  Link B1 : Subsystem
  Link B2 : Subsystem
  Link B3 : Subsystem
  PS-Simulink Converter{1..3,6..7,10..13} (9 alike) : nesl_utility/PS-Simulink Converter  PhysicalDomain=network_engine_domain  SubClassName=ps_output  LeftPortType=input  RightPortType=output  PseudoPeriodic=off  Frequencies=[]  Unit=inherit  AffineConversion=off
  Revolute Joint3 : sm_lib/Joints/Revolute Joint  JointMode=Normal  SenseConstraintForce=off  SenseConstraintForceX=off  SenseConstraintForceY=off  SenseConstraintForceZ=off  SenseConstraintTorque=off  SenseConstraintTorqueX=off  SenseConstraintTorqueY=off  SenseConstraintTorqueZ=off  SenseTotalForce=off  SenseTotalForceX=off  SenseTotalForceY=off  SenseTotalForceZ=off  SenseTotalTorque=off  SenseTotalTorqueX=off  SenseTotalTorqueY=off  SenseTotalTorqueZ=off  CompositeWrenchDir=FollowerOnBase  CompositeWrenchFrame=BaseFrame  EquilibriumPosition=0  EquilibriumPositionUnits=deg  SpringStiffness=0  SpringStiffnessUnits=N*m/deg  DampingCoefficient=fv1  DampingCoefficientUnits=N*m/(rad/s)  TorqueActuationMode=InputTorque  MotionActuationMode=ComputedMotion  SensePosition=on  SenseVelocity=on  SenseAcceleration=on  SenseTorqueForce=off  SenseLowerLimitTorqueForce=off  SenseUpperLimitTorqueForce=off  LowerLimitSpecify=off  LowerLimitBound=-90  LowerLimitBoundUnits=deg  LowerLimitStiffness=1e4  LowerLimitStiffnessUnits=N*m/deg  LowerLimitDamping=10  LowerLimitDampingUnits=N*m/(deg/s)  LowerLimitTransitionRegionWidth=0.1  LowerLimitTransitionRegionWidthUnits=deg  UpperLimitSpecify=off  UpperLimitBound=90  UpperLimitBoundUnits=deg  UpperLimitStiffness=1e4  UpperLimitStiffnessUnits=N*m/deg  UpperLimitDamping=10  UpperLimitDampingUnits=N*m/(deg/s)  UpperLimitTransitionRegionWidth=0.1  UpperLimitTransitionRegionWidthUnits=deg  PositionTargetSpecify=on  PositionTargetPriority=High  PositionTargetValue=th1_0  PositionTargetValueUnits=rad  VelocityTargetSpecify=off  VelocityTargetPriority=High  VelocityTargetValue=0  VelocityTargetValueUnits=deg/s
  Revolute Joint4 : sm_lib/Joints/Revolute Joint  JointMode=Normal  SenseConstraintForce=off  SenseConstraintForceX=off  SenseConstraintForceY=off  SenseConstraintForceZ=off  SenseConstraintTorque=off  SenseConstraintTorqueX=off  SenseConstraintTorqueY=off  SenseConstraintTorqueZ=off  SenseTotalForce=off  SenseTotalForceX=off  SenseTotalForceY=off  SenseTotalForceZ=off  SenseTotalTorque=off  SenseTotalTorqueX=off  SenseTotalTorqueY=off  SenseTotalTorqueZ=off  CompositeWrenchDir=FollowerOnBase  CompositeWrenchFrame=BaseFrame  EquilibriumPosition=0  EquilibriumPositionUnits=deg  SpringStiffness=0  SpringStiffnessUnits=N*m/deg  DampingCoefficient=fv2  DampingCoefficientUnits=N*m/(rad/s)  TorqueActuationMode=InputTorque  MotionActuationMode=ComputedMotion  SensePosition=on  SenseVelocity=on  SenseAcceleration=on  SenseTorqueForce=off  SenseLowerLimitTorqueForce=off  SenseUpperLimitTorqueForce=off  LowerLimitSpecify=off  LowerLimitBound=-90  LowerLimitBoundUnits=deg  LowerLimitStiffness=1e4  LowerLimitStiffnessUnits=N*m/deg  LowerLimitDamping=10  LowerLimitDampingUnits=N*m/(deg/s)  LowerLimitTransitionRegionWidth=0.1  LowerLimitTransitionRegionWidthUnits=deg  UpperLimitSpecify=off  UpperLimitBound=90  UpperLimitBoundUnits=deg  UpperLimitStiffness=1e4  UpperLimitStiffnessUnits=N*m/deg  UpperLimitDamping=10  UpperLimitDampingUnits=N*m/(deg/s)  UpperLimitTransitionRegionWidth=0.1  UpperLimitTransitionRegionWidthUnits=deg  PositionTargetSpecify=on  PositionTargetPriority=High  PositionTargetValue=th2_0  PositionTargetValueUnits=rad  VelocityTargetSpecify=off  VelocityTargetPriority=High  VelocityTargetValue=0  VelocityTargetValueUnits=deg/s
  Revolute Joint5 : sm_lib/Joints/Revolute Joint  JointMode=Normal  SenseConstraintForce=off  SenseConstraintForceX=off  SenseConstraintForceY=off  SenseConstraintForceZ=off  SenseConstraintTorque=off  SenseConstraintTorqueX=off  SenseConstraintTorqueY=off  SenseConstraintTorqueZ=off  SenseTotalForce=off  SenseTotalForceX=off  SenseTotalForceY=off  SenseTotalForceZ=off  SenseTotalTorque=off  SenseTotalTorqueX=off  SenseTotalTorqueY=off  SenseTotalTorqueZ=off  CompositeWrenchDir=FollowerOnBase  CompositeWrenchFrame=BaseFrame  EquilibriumPosition=0  EquilibriumPositionUnits=deg  SpringStiffness=0  SpringStiffnessUnits=N*m/deg  DampingCoefficient=fv3  DampingCoefficientUnits=N*m/(rad/s)  TorqueActuationMode=InputTorque  MotionActuationMode=ComputedMotion  SensePosition=on  SenseVelocity=on  SenseAcceleration=on  SenseTorqueForce=off  SenseLowerLimitTorqueForce=off  SenseUpperLimitTorqueForce=off  LowerLimitSpecify=off  LowerLimitBound=-90  LowerLimitBoundUnits=deg  LowerLimitStiffness=1e4  LowerLimitStiffnessUnits=N*m/deg  LowerLimitDamping=10  LowerLimitDampingUnits=N*m/(deg/s)  LowerLimitTransitionRegionWidth=0.1  LowerLimitTransitionRegionWidthUnits=deg  UpperLimitSpecify=off  UpperLimitBound=90  UpperLimitBoundUnits=deg  UpperLimitStiffness=1e4  UpperLimitStiffnessUnits=N*m/deg  UpperLimitDamping=10  UpperLimitDampingUnits=N*m/(deg/s)  UpperLimitTransitionRegionWidth=0.1  UpperLimitTransitionRegionWidthUnits=deg  PositionTargetSpecify=on  PositionTargetPriority=High  PositionTargetValue=th3_0  PositionTargetValueUnits=rad  VelocityTargetSpecify=off  VelocityTargetPriority=High  VelocityTargetValue=0  VelocityTargetValueUnits=deg/s
  Simulink-PS Converter3 : nesl_utility/Simulink-PS Converter  PhysicalDomain=network_engine_domain  SubClassName=ps_input  LeftPortType=input  RightPortType=output  PseudoPeriodic=off  Frequencies=[]  NoiseDistribution=none  NoiseParameters=[]  Unit=1  AffineConversion=off  FilteringAndDerivatives=provide  SimscapeFilterOrder=1  InputFilterTimeConstant=0.001  UdotUserProvided=0
  Simulink-PS Converter4 : nesl_utility/Simulink-PS Converter  PhysicalDomain=network_engine_domain  SubClassName=ps_input  LeftPortType=input  RightPortType=output  PseudoPeriodic=off  Frequencies=[]  NoiseDistribution=none  NoiseParameters=[]  Unit=1  AffineConversion=off  FilteringAndDerivatives=provide  SimscapeFilterOrder=1  InputFilterTimeConstant=0.001  UdotUserProvided=0
  Simulink-PS Converter5 : nesl_utility/Simulink-PS Converter  PhysicalDomain=network_engine_domain  SubClassName=ps_input  LeftPortType=input  RightPortType=output  PseudoPeriodic=off  Frequencies=[]  NoiseDistribution=none  NoiseParameters=[]  Unit=1  AffineConversion=off  FilteringAndDerivatives=provide  SimscapeFilterOrder=1  InputFilterTimeConstant=0.001  UdotUserProvided=0
  erb115_link5 : Subsystem
  erb145_link1 : Subsystem
  erb145_link3 : Subsystem
  Revolute Joint1 : PMIOPort  Side=Left
  th1B : Outport
  dth1B : Outport  Port=2
  ddth1B : Outport  Port=3
  th2B : Outport  Port=4
  dth2B : Outport  Port=5
  ddth2B : Outport  Port=6
  th3B : Outport  Port=7
  dth3B : Outport  Port=8
  ddth3B : Outport  Port=9
  wires:
  PS-Simulink Converter11/1 -> dth2B/1
  PS-Simulink Converter12/1 -> th3B/1
  PS-Simulink Converter13/1 -> dth3B/1
  tau1B/1 -> Simulink-PS Converter3/1
  tau3B/1 -> Simulink-PS Converter5/1
  tau2B/1 -> Simulink-PS Converter4/1
  PS-Simulink Converter10/1 -> th2B/1
  PS-Simulink Converter6/1 -> th1B/1
  PS-Simulink Converter7/1 -> dth1B/1
  PS-Simulink Converter1/1 -> ddth1B/1
  PS-Simulink Converter2/1 -> ddth2B/1
  PS-Simulink Converter3/1 -> ddth3B/1
  connections:
  PS-Simulink Converter12/LConn1 -- Revolute Joint5/RConn2
  Link B2/RConn1 -- Revolute Joint5/LConn1
  PS-Simulink Converter6/LConn1 -- Revolute Joint3/RConn2
  Revolute Joint4/RConn3 -- PS-Simulink Converter11/LConn1
  Link B1/RConn1 -- Revolute Joint4/LConn1
  Simulink-PS Converter5/RConn1 -- Revolute Joint5/LConn2
  PS-Simulink Converter7/LConn1 -- Revolute Joint3/RConn3
  Simulink-PS Converter4/RConn1 -- Revolute Joint4/LConn2
  Link B1/LConn1 -- Revolute Joint3/RConn1
  Link B2/LConn1 -- erb145_link3/RConn1
  Revolute Joint5/RConn3 -- PS-Simulink Converter13/LConn1
  erb115_link5/LConn1 -- Revolute Joint5/RConn1
  Simulink-PS Converter3/RConn1 -- Revolute Joint3/LConn2
  PS-Simulink Converter10/LConn1 -- Revolute Joint4/RConn2
  PS-Simulink Converter1/LConn1 -- Revolute Joint3/RConn4
  PS-Simulink Converter2/LConn1 -- Revolute Joint4/RConn4
  PS-Simulink Converter3/LConn1 -- Revolute Joint5/RConn4
  erb145_link1/RConn1 -- Revolute Joint3/LConn1
  erb145_link1/LConn1 -- Revolute Joint1/RConn1
  erb145_link3/LConn1 -- Revolute Joint4/RConn1
  Link B3/LConn1 -- erb115_link5/RConn1

== system redundancy/Full system (planar version)/cables ==
  Inertia : sm_lib/Body Elements/Inertia  InertiaType=Custom  Mass=m_cables  MassUnits=kg  CenterOfMass=[0, 0, 0]  CenterOfMassUnits=m  MomentsOfInertia=[0.0416667, 90.0025, 90.0025]  MomentsOfInertiaUnits=kg*m^2  ProductsOfInertia=[0 0 0]  ProductsOfInertiaUnits=kg*m^2  GraphicType=None  MarkerShape=Inertia  MarkerSize=20  GraphicVisPropType=SimpleVisualProperties  GraphicDiffuseColor=[0.5 0.5 0.5]  GraphicSpecularColor=[0.5 0.5 0.5 1.0]  GraphicAmbientColor=[0.15 0.15 0.15 1.0]  GraphicEmissiveColor=[0.0 0.0 0.0 1.0]  GraphicShininess=75  GraphicOpacity=1.0
  InertiaOriginTransform : sm_lib/Frames and Transforms/Rigid Transform  TranslationMethod=None  TranslationStandardOffset=0  TranslationLengthUnit=m  TranslationStandardAxis=+Z  TranslationCartesianOffset=inertial_disp_cables  TranslationROffset=0  TranslationROffsetUnits=m  TranslationZOffset=0  TranslationZOffsetUnits=m  TranslationThetaOffset=0  TranslationThetaOffsetUnits=deg  RotationMethod=None  RotationAngleUnits=deg  RotationStandardAxis=+Z  RotationAngle=0.0  RotationArbitraryAxis=[0 0 1]  FollAlignAxisA=+X  BaseAlignAxisA=+Y  FollAlignAxisB=+Y  BaseAlignAxisB=+Z  RotationSequenceAxes=BaseAxes  RotationSequence=XYZ  RotationSequenceAngles=[0, 0, 0]  RotationSequenceAnglesUnits=rad  RotationMatrix=[1 0 0; 0 1 0; 0 0 1]
  ReferenceFrame : sm_lib/Frames and Transforms/Reference Frame
  Rigid Transform : sm_lib/Frames and Transforms/Rigid Transform  TranslationMethod=StandardAxis  TranslationStandardOffset=L/2  TranslationLengthUnit=m  TranslationStandardAxis=-X  TranslationCartesianOffset=[0 0 0]  TranslationROffset=0  TranslationROffsetUnits=m  TranslationZOffset=0  TranslationZOffsetUnits=m  TranslationThetaOffset=0  TranslationThetaOffsetUnits=deg  RotationMethod=None  RotationAngleUnits=deg  RotationStandardAxis=+Z  RotationAngle=0.0  RotationArbitraryAxis=[0 0 1]  FollAlignAxisA=+X  BaseAlignAxisA=+Y  FollAlignAxisB=+Y  BaseAlignAxisB=+Z  RotationSequenceAxes=FollowerAxes  RotationSequence=XYX  RotationSequenceAngles=[0 0 0]  RotationSequenceAnglesUnits=deg  RotationMatrix=[1 0 0; 0 1 0; 0 0 1]
  Rigid Transform1 : sm_lib/Frames and Transforms/Rigid Transform  TranslationMethod=StandardAxis  TranslationStandardOffset=L/2  TranslationLengthUnit=m  TranslationStandardAxis=+X  TranslationCartesianOffset=[0 0 0]  TranslationROffset=0  TranslationROffsetUnits=m  TranslationZOffset=0  TranslationZOffsetUnits=m  TranslationThetaOffset=0  TranslationThetaOffsetUnits=deg  RotationMethod=StandardAxis  RotationAngleUnits=deg  RotationStandardAxis=+Z  RotationAngle=90  RotationArbitraryAxis=[0 0 1]  FollAlignAxisA=+X  BaseAlignAxisA=+Y  FollAlignAxisB=+Y  BaseAlignAxisB=+Z  RotationSequenceAxes=FollowerAxes  RotationSequence=XYX  RotationSequenceAngles=[0 0 0]  RotationSequenceAnglesUnits=deg  RotationMatrix=[1 0 0; 0 1 0; 0 0 1]
  Visual : sm_lib/Body Elements/File Solid  ExtGeomFileName=cables_new_new.stl  UnitType=Custom  ExtGeomFileUnits=m  StepReaderType=HEX  ExportConvexHullGeometry=off  InertiaType=Custom  Mass=0  MassUnits=kg  CenterOfMass=[0, 0, 0]  CenterOfMassUnits=m  MomentsOfInertia=[0, 0, 0]  MomentsOfInertiaUnits=kg*m^2  ProductsOfInertia=[0, 0, 0]  ProductsOfInertiaUnits=kg*m^2  BasedOnType=DensityFromFile  Density=1000  DensityUnits=kg/m^3  DoExposeReferenceFrame=on  SerializedFrames=<Frames/>  GraphicType=FromGeometry  MarkerShape=Sphere  MarkerSize=10  GraphicVisPropType=SimpleVisualProperties  GraphicDiffuseColor=[0.4 0.4 0.4]  GraphicSpecularColor=[0.5 0.5 0.5 1.0]  GraphicAmbientColor=[0.15 0.15 0.15 1.0]  GraphicEmissiveColor=[0.0 0.0 0.0 1.0]  GraphicShininess=75  GraphicOpacity=1
  VisualOriginTransform : sm_lib/Frames and Transforms/Rigid Transform  TranslationMethod=Cartesian  TranslationStandardOffset=0  TranslationLengthUnit=m  TranslationStandardAxis=+Z  TranslationCartesianOffset=[L/2, 0, 0]  TranslationROffset=0  TranslationROffsetUnits=m  TranslationZOffset=0  TranslationZOffsetUnits=m  TranslationThetaOffset=0  TranslationThetaOffsetUnits=deg  RotationMethod=StandardAxis  RotationAngleUnits=deg  RotationStandardAxis=+Y  RotationAngle=90  RotationArbitraryAxis=[0 0 1]  FollAlignAxisA=+X  BaseAlignAxisA=+Y  FollAlignAxisB=+Y  BaseAlignAxisB=+Z  RotationSequenceAxes=BaseAxes  RotationSequence=XYZ  RotationSequenceAngles=[135, 0, 0]  RotationSequenceAnglesUnits=deg  RotationMatrix=[1 0 0; 0 1 0; 0 0 1]
  VisualOriginTransform1 : sm_lib/Frames and Transforms/Rigid Transform  TranslationMethod=None  TranslationStandardOffset=0  TranslationLengthUnit=m  TranslationStandardAxis=+Z  TranslationCartesianOffset=[1.58, 0, 0]  TranslationROffset=0  TranslationROffsetUnits=m  TranslationZOffset=0  TranslationZOffsetUnits=m  TranslationThetaOffset=0  TranslationThetaOffsetUnits=deg  RotationMethod=StandardAxis  RotationAngleUnits=deg  RotationStandardAxis=+Z  RotationAngle=180  RotationArbitraryAxis=[0 0 1]  FollAlignAxisA=+X  BaseAlignAxisA=+Y  FollAlignAxisB=+Y  BaseAlignAxisB=+Z  RotationSequenceAxes=BaseAxes  RotationSequence=XYZ  RotationSequenceAngles=[135, 0, 0]  RotationSequenceAnglesUnits=deg  RotationMatrix=[1 0 0; 0 1 0; 0 0 1]
  B : PMIOPort  Side=Left
  F : PMIOPort  Port=2  Side=Right
  connections:
  Inertia/RConn1 -- InertiaOriginTransform/RConn1
  InertiaOriginTransform/LConn1 -- VisualOriginTransform1/LConn1 -- ReferenceFrame/RConn1 -- Rigid Transform1/LConn1 -- Rigid Transform/LConn1
  Visual/RConn1 -- VisualOriginTransform/RConn1
  Rigid Transform/RConn1 -- B/RConn1
  F/RConn1 -- Rigid Transform1/RConn1
  VisualOriginTransform1/RConn1 -- VisualOriginTransform/LConn1
